simulink model "sim_aircraft_3d_animation"  (R2020b)
settings: Solver=VariableStepAuto  StartTime=0.0  StopTime=10.0  RelTol=1e-3
settings Model: Creator=seanb  LastModifiedBy=seanb

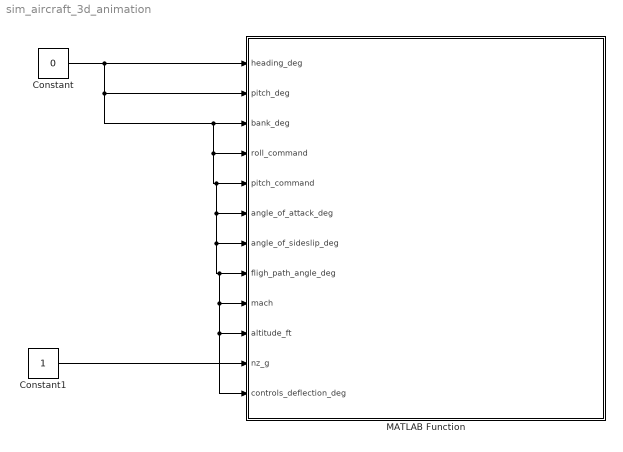
== system sim_aircraft_3d_animation ==
  Constant : Constant  Value=0
  Constant1 : Constant
  MATLAB Function : MATLAB Function  TreatAsAtomicUnit=on
  wires:
  Constant/1 -> MATLAB Function/12(controls_deflection_deg), MATLAB Function/10(altitude_ft), MATLAB Function/9(mach), MATLAB Function/8(fligh_path_angle_deg), MATLAB Function/7(angle_of_sideslip_deg), MATLAB Function/6(angle_of_attack_deg), MATLAB Function/5(pitch_command), MATLAB Function/4(roll_command), MATLAB Function/3(bank_deg), MATLAB Function/2(pitch_deg), MATLAB Function/1(heading_deg)
  Constant1/1 -> MATLAB Function/11(nz_g)

== matlab function sim_aircraft_3d_animation/MATLAB Function ==
  data: heading_deg input; pitch_deg input; bank_deg input; roll_command input; pitch_command input; angle_of_attack_deg input; angle_of_sideslip_deg input; fligh_path_angle_deg input; mach input; altitude_ft input; nz_g input; controls_deflection_deg input; animation_init_struct parameter
function aircraft_3d_animation_update(...
    heading_deg,...
    pitch_deg,...
    bank_deg,...
    roll_command,...
    pitch_command,...
    angle_of_attack_deg,...
    angle_of_sideslip_deg,...
    fligh_path_angle_deg,...   
    mach,...                   
    altitude_ft,...            
    nz_g,...                  
    controls_deflection_deg,...
    animation_init_struct)

%Dont know if it is running, neet to create initialization script and finish simulink model

    % Pitch disc
    M = makehgtform('zrotate', -heading_deg* pi / 180);      % Heading rotation
    set(animation_init_struct.euler_hgt(3), 'Matrix', M)
    
    % Roll disc
    M1 = makehgtform('zrotate',  -heading_deg * pi / 180);   % Heading rotation
    M2 = makehgtform('yrotate', pitch_deg * pi / 180);   % Pitch rotation
    set(animation_init_struct.euler_hgt(2), 'Matrix', M1 * M2)
    
    % Roll line
    M = makehgtform('xrotate', -bank_deg * pi / 180);
    set(animation_init_struct.euler_hgt(5), 'Matrix', M)
    
    % Pitch line
    M = makehgtform('yrotate', pitch_deg * pi / 180);
    set(animation_init_struct.euler_hgt(6), 'Matrix', M)
    
    % Heading line
    M = makehgtform('zrotate', -heading_deg * pi / 180);
    set(animation_init_struct.euler_hgt(7), 'Matrix', M)
    
    % AIRCRAFT BODY
    M1 = makehgtform('zrotate',  -heading_deg * pi / 180);  % Heading rotation
    M2 = makehgtform('yrotate', pitch_deg * pi / 180);  % Pitch rotation
    M3 = makehgtform('xrotate', -bank_deg * pi / 180);  % bank_deg rotation
    set(AV_hg, 'Matrix',M1 * M2 * M3)
    
    % controls_deflection_deg
    for j=1:length(Model3D.Control)
        M1 = makehgtform('translate', -Model3D.Control(j).rot_point);   % Heading
        M2 = makehgtform('axisrotate', Model3D.Control(j).rot_vect, controls_deflection_deg(j) * pi / 180);  % Pitch
        M3 = makehgtform('translate', Model3D.Control(j).rot_point);  % bank_deg
        set(CONT_hg(j), 'Matrix', M3 * M2 * M1);
    end
    
    % Compute Aerodynamic Speed Vector
    Lbh_i = Lbh(heading_deg, pitch_deg, bank_deg);
    Vaer  = Lbh_i' * Lbw(angle_of_attack_deg, angle_of_sideslip_deg) * [AC_DIMENSION; 0; 0];
    X_aer = [0, -Vaer(1)];
    Y_aer = [0, +Vaer(2)];
    Z_aer = [0, -Vaer(3)];
    
    n_p = 10;
    Vaer_angle_of_sideslip0 = zeros(n_p, 3);
    for ik = 1:n_p
        Vaer_angle_of_sideslip0(ik, :) = Lbh_i' * Lbw(angle_of_attack_deg, angle_of_sideslip_deg * (ik - 1) / (n_p - 1)) * [AC_DIMENSION; 0; 0];
    end
    X_aer_angle_of_sideslip0 = [0, -Vaer_angle_of_sideslip0(:, 1)'];
    Y_aer_angle_of_sideslip0 = [0, +Vaer_angle_of_sideslip0(:, 2)'];
    Z_aer_angle_of_sideslip0 = [0, -Vaer_angle_of_sideslip0(:, 3)'];
    
    Vaer_angle_of_attack0angle_of_sideslip0 = zeros(n_p, 3);
    for ik=1:n_p
        Vaer_angle_of_attack0angle_of_sideslip0(ik, :)=Lbh_i'*Lbw(angle_of_attack_deg*(ik-1)/(n_p-1),0)*[AC_DIMENSION;0;0];
    end
    X_aer_angle_of_attack0angle_of_sideslip0 = [0, -Vaer_angle_of_attack0angle_of_sideslip0(:, 1)'];
    Y_aer_angle_of_attack0angle_of_sideslip0 = [0, +Vaer_angle_of_attack0angle_of_sideslip0(:, 2)'];
    Z_aer_angle_of_attack0angle_of_sideslip0 = [0, -Vaer_angle_of_attack0angle_of_sideslip0(:, 3)'];
    
    refreshdata(hdle_aero, 'caller')
    refreshdata(hdle_aero_angle_of_sideslip0, 'caller')
    refreshdata(hdle_aero_angle_of_attack0angle_of_sideslip0, 'caller')
    
    set(hdle_text_t, 'String',sprintf('t= %3.2f sec',(i-1)*frame_time*speedx))
    set(hdle_text_valtitude, 'String',strcat(num2str(mach, '%1.2f'), 'M @ ',num2str(altitude_ft/0.3048, '%4.0fft')))
    set(hdle_text_psi_deg, 'String',strcat('\psi=',num2str(heading_deg, '%2.1f'), 'deg'))
    set(hdle_text_th, 'String',strcat('\theta=',num2str(pitch_deg, '%2.1f'), 'deg'))
    set(hdle_text_phi, 'String',strcat('\phi=',num2str(bank_deg, '%2.1f'), 'deg'))
    set(hdle_text_angle_of_attack, 'String',strcat('\alpha=',num2str(angle_of_attack_deg, '%2.1f'), 'deg'))
    
    % Change the aircraft's body color when the airflow incidence angles exceed the limits (change as you wish)
    max_aos = 15; % [deg]
    max_aoa = 40; % [deg]
    max_nz  = 10; % [g]
    if abs(angle_of_sideslip_deg) < max_aos && angle_of_attack_deg < max_aoa
        FontWeight = 'NORMAL';
        set(AV(1), 'FaceColor', Model3D.Aircraft(1).color);
    else
        FontWeight = 'BOLD';
        set(AV(1), 'FaceColor', [1.0 0.4 0.4]);
    end
    TextColor = (abs(angle_of_sideslip_deg) < max_aos) .* text_color + (abs(angle_of_sideslip_deg) >= max_aos) * [1, 0, 0];
    set(hdle_text_angle_of_sideslip, 'String', strcat('\beta=', num2str(angle_of_sideslip_deg, '%2.1f'), 'deg'), 'Color', TextColor, 'FontWeight', FontWeight)
    set(hdle_text_gam, 'String', strcat('\gamma=', num2str(fligh_path_angle_deg, '%2.1f'), 'deg'))
    if nz_g < max_nz
        FontWeight = 'NORMAL';
    else
        FontWeight = 'BOLD';
    end
    TextColor = (nz_g < max_nz) .* text_color + (nz_g >= max_nz) * [1, 0, 0];
    set(hdle_text_nz, 'String', strcat('N_z=', num2str(nz_g, '%2.1f'), 'g'), 'Color', TextColor, 'FontWeight', FontWeight)
    
    % Detect control surfaces saturations
    idx_sat = controls_deflection_deg(:) >= max_deflection(2, :)*0.99 | controls_deflection_deg(:) <= max_deflection(:)*0.99;
    idx_nosat = ~idx_sat;
    set(CONT(idx_sat), 'FaceColor', 'y');
    set(CONT(idx_nosat), 'FaceColor', Model3D.Control(1).color);
    
    % Stick Position
    STICK_X     = [0 -roll_command];
    STICK_X_END = -roll_command;
    STICK_Y     = min(1,[0 (1.0/0.6.*max(0,pitch_command)+min(0,pitch_command))]);
    STICK_Y_END = min(1,(1.0/0.6.*max(0,pitch_command)+min(0,pitch_command)));
    XSTICK         = -roll_command;
    YSTICK         = min(1,(1.0 / 0.6 .* max(0, pitch_command) + min(0, pitch_command)));
    
    % Refresh stick position plot
    refreshdata(h_stick1, 'caller')
    refreshdata(h_stick2, 'caller')
    refreshdata(h_stick3, 'caller')
    
    % Real-time
    drawnow;
end

function Lbh = Lbh(heading_deg, pitch_deg, phi)
% Rotation matrix from NED axis to Aircraft's body axis
sps = sind(heading_deg);
cps = cosd(heading_deg);
sth = sind(pitch_deg);
cth = cosd(pitch_deg);
sph = sind(phi);
cph = cosd(phi);
Lb1 = [...
    1   0   0
    0   cph sph
    0  -sph cph];
L12 = [...
    cth 0   -sth
    0   1   0
    sth 0   cth];
L2h = [...
    cps sps 0
    -sps cps 0
    0   0   1];
Lbh = Lb1 * L12 * L2h;
end

function Lbw = Lbw(angle_of_attack, angle_of_sideslip)
% Rotation matrix from Wind-axis to Aircraft's body axis
sa = sind(angle_of_attack);
ca = cosd(angle_of_attack);
sb = sind(angle_of_sideslip);
cb = cosd(angle_of_sideslip);
Lbw = [...
    ca*cb -ca*sb -sa
    sb cb 0
    sa*cb -sa*sb ca];
end
